simulink model "Simulink2"  (Simulink 5.0)
settings: Solver=ode45  StartTime=0.0  StopTime=50.0  RelTol=1e-3
settings Model: LastModifiedBy=stevel

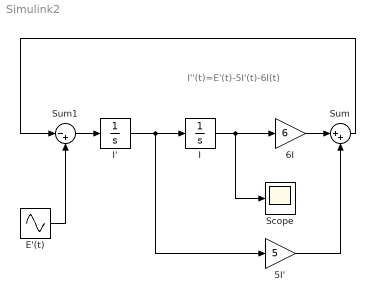
== system Simulink2 ==
  note: I''(t)=E'(t)-5I'(t)-6I(t)
  5I' : Gain  Gain=5  SaturateOnIntegerOverflow=on
  6I : Gain  Gain=6  SaturateOnIntegerOverflow=on
  E'(t) : Sin  Amplitude=10  SampleTime=0
  I : Integrator  InitialCondition=1
  I' : Integrator  InitialCondition=5
  Scope : Scope
  Sum : Sum  Inputs=|++  SaturateOnIntegerOverflow=on
  Sum1 : Sum  Inputs=|-+  SaturateOnIntegerOverflow=on
  wires:
  I'/1 -> I/1, 5I'/1
  I/1 -> 6I/1, Scope/1
  6I/1 -> Sum/1
  Sum1/1 -> I'/1
  E'(t)/1 -> Sum1/2
  5I'/1 -> Sum/2
  Sum/1 -> Sum1/1
